simulink model "test_IO_block_function"  (R2016b)
settings: Solver=ode45  StartTime=0.0  StopTime=50  RelTol=1e-3
undefined symbols (not defined in the file or in its folder): car, car_init
libraries: realtime_pacer_lib x2
settings Model: Creator=ciba  LastModifiedBy=ciba
settings DataIOCC: LimitDataPoints=on  SaveFormat=Array  SignalLoggingSaveFormat=ModelDataLogs
settings OptimizationCC: DefaultParameterBehavior=Inlined  UseDivisionForNetSlopeComputation=on  UseFloatMulNetSlope=on  InlineInvariantSignals=on  PassReuseOutputArgsAs=Individual arguments  ZeroExternalMemoryAtStartup=off  ZeroInternalMemoryAtStartup=off  NoFixptDivByZeroProtection=on  EfficientFloat2IntCast=on  LifeSpan=1
settings DebuggingCC: SaveWithParameterizedLinksMsg=none  SignalResolutionControl=TryResolveAllWithWarning  MultiTaskDSMMsg=warning  MultiTaskCondExecSysMsg=none  ParameterTunabilityLossMsg=error  SFUnexpectedBacktrackingDiag=warning  SFNoUnconditionalDefaultTransitionDiag=warning  SFExecutionAtInitializationDiag=none
settings HardwareCC: TargetBitPerPointer=64  TargetBitPerSizeT=64  TargetBitPerPtrDiffT=64  TargetLongLongMode=on  TargetIntDivRoundTo=Zero  TargetEndianess=LittleEndian  TargetWordSize=64  TargetHWDeviceType=MATLAB Host  ProdEqTarget=off
settings ModelReferenceCC: PropagateSignalLabelsOutOfModel=off
settings RTWCC: SystemTargetFile=ert.tlc  TemplateMakefile=ert_default_tmf  Description=Embedded Coder  GenerateReport=on  IncludeHyperlinkInReport=on  LaunchReport=on  GenerateTraceInfo=on  GenerateTraceReport=on  GenerateTraceReportSl=on  GenerateTraceReportSf=on  GenerateTraceReportEml=on  GenerateCodeMetricsReport=on
settings CodeAppCC: ForceParamTrailComments=on  IgnoreCustomStorageClasses=off  OperatorAnnotations=on  SimulinkDataObjDesc=on  SFDataObjDesc=on  MATLABFcnDesc=on  CustomSymbolStrGlobalVar=rt$N$M  CustomSymbolStrType=$N$M  CustomSymbolStrFcn=$N$M$F  CustomSymbolStrMacro=$N$M  InsertBlockDesc=on  MATLABSourceComments=on
settings ERTTargetCC: GenerateSampleERTMain=on  CombineSignalStateStructs=on  SupportComplex=off  SupportContinuousTime=on  SupportNonInlinedSFcns=on  InlinedParameterPlacement=NonHierarchical  ERTCustomFileTemplate=example_file_process.tlc  ERTFilePackagingFormat=CompactWithDataFile
settings ConfigComp: CovMetricSettings=dw  CovHtmlReporting=on  CovSaveCumulativeToWorkspaceVar=on  CovSaveSingleToWorkspaceVar=on  CovExternalEMLEnable=off

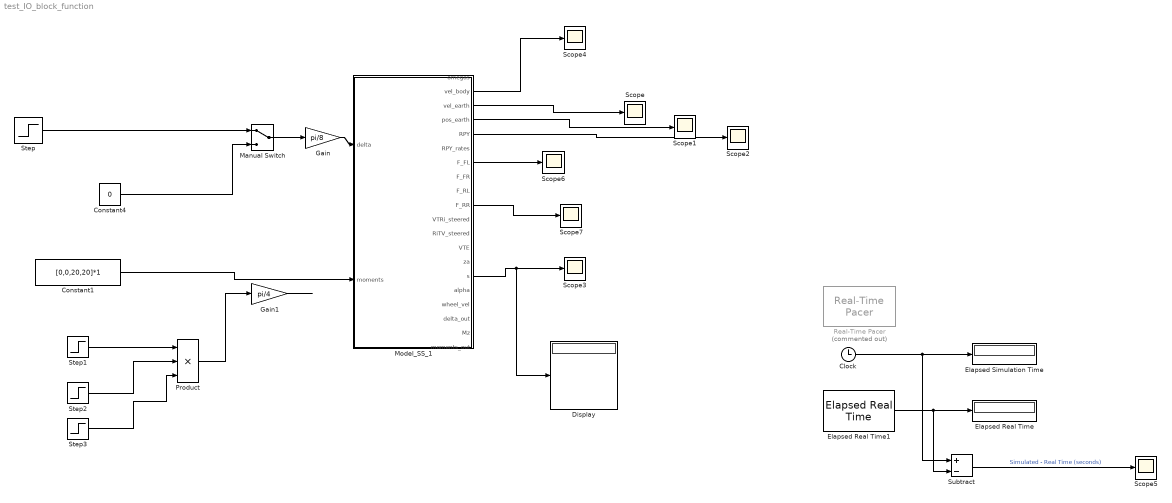
== system test_IO_block_function ==
  Clock : Clock
  Constant1 : Constant  Value=[0,0,20,20]*1
  Constant4 : Constant  Value=0
  Display : Display
  Elapsed Real Time : Display
      settings: Decimation=2
  Elapsed Real Time1 : realtime_pacer_lib/Elapsed Real Time
  Elapsed Simulation Time : Display
      settings: Decimation=2
  Gain : Gain  Gain=pi/8
  Gain1 : Gain  Gain=pi/4
  Manual Switch : ManualSwitch
  Model_SS_1 : Subsystem
  Product : Product  Inputs=3
  Real-Time Pacer : realtime_pacer_lib/Real-Time Pacer  Commented=on  simTimePerRealTime=1
  Scope{,1..7} (8 alike) : Scope
  Step : Step  Time=5  SampleTime=0
  Step1 : Step  Time=0  SampleTime=0
  Step2 : Step  Time=10  SampleTime=0
  Step3 : Step  Time=20  Before=1  After=-1  SampleTime=0
  Subtract : Sum  Inputs=+-
  wires:
  Step/1 -> Manual Switch/1
  Constant4/1 -> Manual Switch/2
  Manual Switch/1 -> Gain/1
  Model_SS_1/3(vel_earth) -> Scope/1
  Model_SS_1/4(pos_earth) -> Scope1/1
  Model_SS_1/5(RPY) -> Scope2/1
  Gain/1 -> Model_SS_1/1(delta)
  Model_SS_1/15(s) -> Display/1, Scope3/1
  Step2/1 -> Product/2
  Step1/1 -> Product/1
  Step3/1 -> Product/3
  Gain1/1 -> ?
  Product/1 -> Gain1/1
  Clock/1 -> Elapsed Simulation Time/1, Subtract/1
  Subtract/1 -> Scope5/1  "Simulated - Real Time (seconds)"
  Elapsed Real Time1/1 -> Elapsed Real Time/1, Subtract/2
  Model_SS_1/2(vel_body) -> Scope4/1
  Model_SS_1/7(F_FL) -> Scope6/1
  Model_SS_1/10(F_RR) -> Scope7/1
  Constant1/1 -> Model_SS_1/2("moments ")

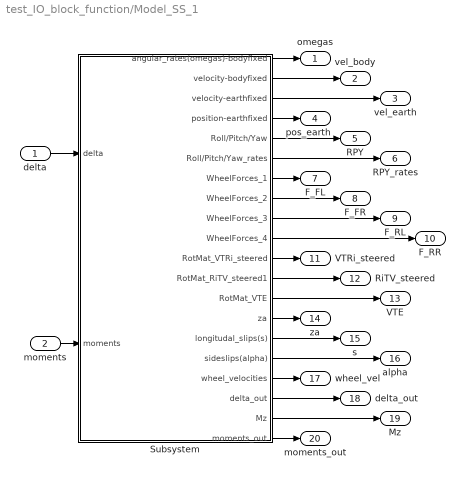
== system test_IO_block_function/Model_SS_1 ==
  delta : Inport
  "moments " : Inport  Port=2  PortDimensions=4
  Subsystem : Subsystem
  omegas : Outport
  vel_body : Outport  Port=2
  vel_earth : Outport  Port=3
  pos_earth : Outport  Port=4
  RPY : Outport  Port=5
  RPY_rates : Outport  Port=6
  F_FL : Outport  Port=7
  F_FR : Outport  Port=8
  F_RL : Outport  Port=9
  F_RR : Outport  Port=10
  VTRi_steered : Outport  Port=11
  RiTV_steered : Outport  Port=12
  VTE : Outport  Port=13
  za : Outport  Port=14
  s : Outport  Port=15
  alpha : Outport  Port=16
  wheel_vel : Outport  Port=17
  delta_out : Outport  Port=18
  Mz : Outport  Port=19
  moments_out : Outport  Port=20
  wires:
  Subsystem/20(moments_out) -> moments_out/1
  Subsystem/19(Mz) -> Mz/1
  Subsystem/18(delta_out) -> delta_out/1
  Subsystem/17(wheel_velocities) -> wheel_vel/1
  Subsystem/16(sideslips(alpha)) -> alpha/1
  Subsystem/15(longitudal_slips(s)) -> s/1
  Subsystem/14(za) -> za/1
  Subsystem/13(RotMat_VTE) -> VTE/1
  Subsystem/12(RotMat_RiTV_steered1) -> RiTV_steered/1
  Subsystem/11(RotMat_VTRi_steered) -> VTRi_steered/1
  Subsystem/10(WheelForces_4) -> F_RR/1
  Subsystem/9(WheelForces_3) -> F_RL/1
  Subsystem/8(WheelForces_2) -> F_FR/1
  Subsystem/7(WheelForces_1) -> F_FL/1
  Subsystem/6(Roll/Pitch/Yaw_rates) -> RPY_rates/1
  Subsystem/5(Roll/Pitch/Yaw) -> RPY/1
  Subsystem/4(position-earthfixed) -> pos_earth/1
  Subsystem/3(velocity-earthfixed) -> vel_earth/1
  Subsystem/2(velocity-bodyfixed) -> vel_body/1
  Subsystem/1(angular_rates(omegas)-bodyfixed) -> omegas/1
  "moments "/1 -> Subsystem/2(moments)
  delta/1 -> Subsystem/1(delta)

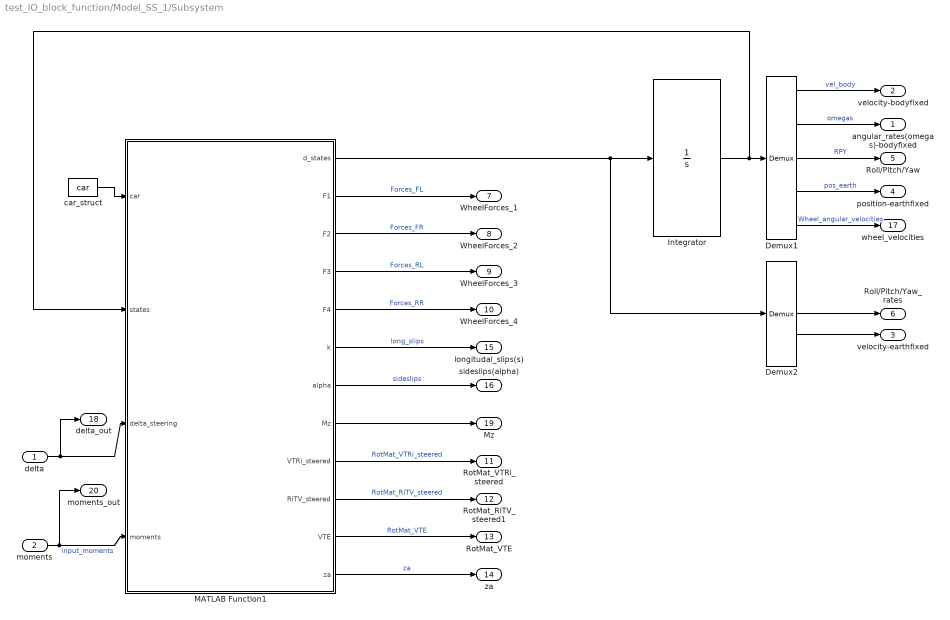
== system test_IO_block_function/Model_SS_1/Subsystem ==
  delta : Inport
  moments : Inport  Port=2
  Demux1 : Demux  Outputs=[3,3,3,3,4]
  Demux2 : Demux  Outputs=[3,3,3,3,4]
  Integrator : Integrator  InitialCondition=car_init
  MATLAB Function1 : MATLAB Function  TreatAsAtomicUnit=on
  car_struct : Constant  Value=car  OutDataTypeStr=Bus: car_bus
  angular_rates(omegas)-bodyfixed : Outport  PortDimensions=3
  velocity-bodyfixed : Outport  Port=2  PortDimensions=3
  velocity-earthfixed : Outport  Port=3  PortDimensions=3
  position-earthfixed : Outport  Port=4  PortDimensions=3
  Roll/Pitch/Yaw : Outport  Port=5  PortDimensions=3
  Roll/Pitch/Yaw_rates : Outport  Port=6  PortDimensions=3
  WheelForces_1 : Outport  Port=7
  WheelForces_2 : Outport  Port=8
  WheelForces_3 : Outport  Port=9
  WheelForces_4 : Outport  Port=10
  RotMat_VTRi_steered : Outport  Port=11
  RotMat_RiTV_steered1 : Outport  Port=12
  RotMat_VTE : Outport  Port=13
  za : Outport  Port=14
  longitudal_slips(s) : Outport  Port=15
  sideslips(alpha) : Outport  Port=16
  wheel_velocities : Outport  Port=17
  delta_out : Outport  Port=18
  Mz : Outport  Port=19
  moments_out : Outport  Port=20
  wires:
  Demux1/5 -> wheel_velocities/1  "Wheel_angular_velocities"
  MATLAB Function1/5(F4) -> WheelForces_4/1  "Forces_RR"
  MATLAB Function1/3(F2) -> WheelForces_2/1  "Forces_FR"
  MATLAB Function1/2(F1) -> WheelForces_1/1  "Forces_FL"
  MATLAB Function1/4(F3) -> WheelForces_3/1  "Forces_RL"
  MATLAB Function1/11(VTE) -> RotMat_VTE/1  "RotMat_VTE"
  delta/1 -> MATLAB Function1/3(delta_steering), delta_out/1
  MATLAB Function1/7(alpha) -> sideslips(alpha)/1  "sideslips"
  MATLAB Function1/6(k) -> longitudal_slips(s)/1  "long_slips"
  Demux1/3 -> Roll/Pitch/Yaw/1  "RPY"
  MATLAB Function1/9(VTRi_steered) -> RotMat_VTRi_steered/1  "RotMat_VTRi_steered"
  Demux1/2 -> angular_rates(omegas)-bodyfixed/1  "omegas"
  Demux1/4 -> position-earthfixed/1  "pos_earth"
  Demux1/1 -> velocity-bodyfixed/1  "vel_body"
  MATLAB Function1/12(za) -> za/1  "za"
  moments/1 -> moments_out/1, MATLAB Function1/4(moments)  "input_moments"
  MATLAB Function1/10(RiTV_steered) -> RotMat_RiTV_steered1/1  "RotMat_RiTV_steered"
  MATLAB Function1/1(d_states) -> Demux2/1, Integrator/1
  Integrator/1 -> MATLAB Function1/2(states), Demux1/1
  car_struct/1 -> MATLAB Function1/1(car)
  MATLAB Function1/8(Mz) -> Mz/1
  Demux2/4 -> velocity-earthfixed/1
  Demux2/3 -> Roll/Pitch/Yaw_rates/1

== matlab function test_IO_block_function/Model_SS_1/Subsystem/MATLAB Function1 ==
  data: car input Bus: car_bus; d_states output size=16; states input size=16; delta_steering input size=1; F1 output size=3; F2 output size=3; F3 output size=3; F4 output size=3; k output size=4; alpha output size=4; Mz output size=4; VTRi_steered output size=[3,3]; RiTV_steered output size=[3,3]; VTE output size=[3,3]; za output size=4; moments input size=4
function [ d_states,F1,F2,F3,F4,k,alpha,Mz,VTRi_steered,RiTV_steered,VTE,za ] ...
    = tiresBody( car,states,delta_steering,moments )

[ d_states,F_R,k,alpha,Mz,VTRi_steered,RiTV_steered,VTE,za ] ...
    = tires_and_body( car,states,delta_steering,moments );

F1 = F_R(:,1);
F2 = F_R(:,2);
F3 = F_R(:,3);
F4 = F_R(:,4);
